simulink model "Discrete_Bicycle_Simulink_Model"  (R2024a)
settings: Solver=ode4  StartTime=0.0  StopTime=100  FixedStep=0.01  RelTol=1e-3
undefined symbols (not defined in the file): Ad, Aobs, Bd, Bobs, c, Cd, Cobs, Dd, Dobs, Kd, lambda, Ts, v, w, x0, xhat0
settings Model: Creator=Vipuls  LastModifiedBy=Vipuls

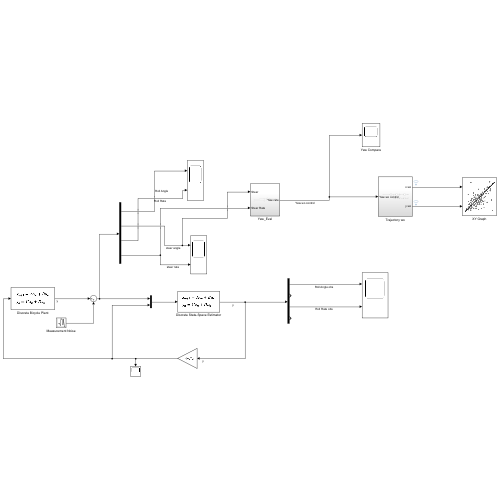
[thumbnail: Simulink's stored preview of the top-level diagram]
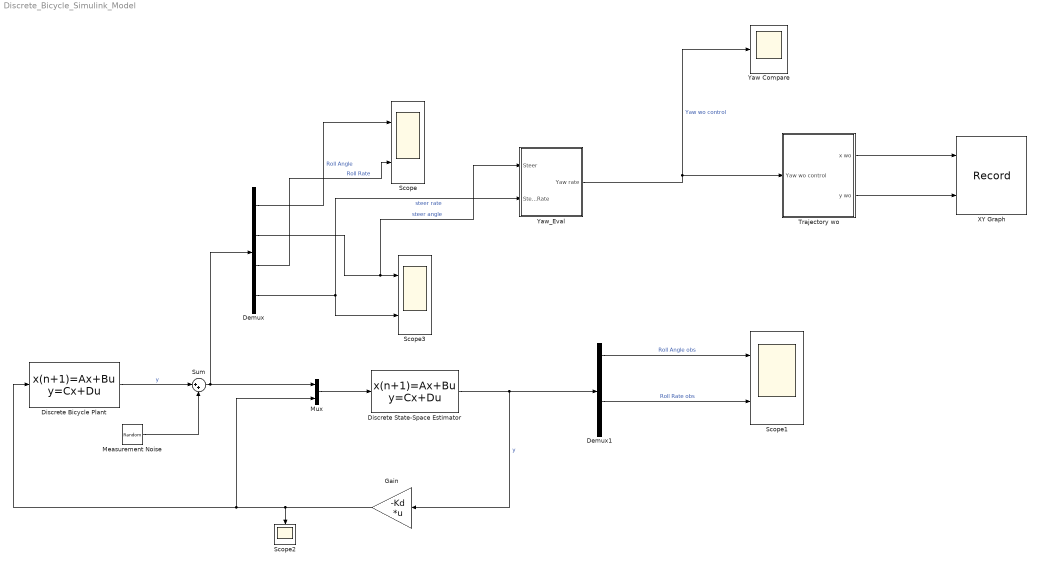
== system Discrete_Bicycle_Simulink_Model ==
  Demux : Demux
  Demux1 : Demux
  Discrete Bicycle Plant : DiscreteStateSpace  A=Ad  B=Bd  C=Cd  D=Dd  InitialCondition=x0  SampleTime=Ts
  Discrete State-Space Estimator : DiscreteStateSpace  A=Aobs  B=Bobs  C=Cobs  D=Dobs  InitialCondition=xhat0  SampleTime=-1
  Gain : Gain  Gain=-Kd  Multiplication=Matrix(K*u)
  Measurement Noise : RandomNumber  Variance=[0.0001, 0.0001, 0.0001, 0.0001]  SampleTime=Ts
  Mux : Mux  Inputs=2
  Scope : Scope  NumInputPorts=2
  Scope1 : Scope  NumInputPorts=2
  Scope2 : Scope
  Scope3 : Scope  NumInputPorts=2
  Sum : Sum  Inputs=|++
  Trajectory wo : Subsystem
  XY Graph : Record  FileSettingsInternal="{\"entries\":[{\"content\":{\"excelSettings\":{\"content\":{},\"type\":\"Streamout.ExcelSettings\"}},\"type\":\"Streamout.FileSettingStorage\",\"uuid\":\"\"}],\"packageUris\":[\"http:\\/\\/schema.mathworks.com\\/mf0\\/streamout_blocks\\/R2020a\"],\"version\":\"1.0\"}"  Layout=[1 1]  SignalsInternal="{\"entries\":[{\"content\":{\"signals\":[{\"content\":{\"blockPath\":[],\"dimensions\":[1],\"domain\":\"\",\"lineColor\":\"#0072bd\",\"lineWidth\":2,\"plots\":[ 1 ],\"port\":1,\"sid\":[\"\"],\"signalID\":1,\"signalName\":\"Trajectory wo:1\"},\"type\":\"RecordBlkView.Signal\",\"uuid\":\"\"},{\"content\":{\"blockPath\":[],\"dimensions\":[1],\"domain\":\"\",\"lineColor\":\"#d95319\",\"lineWidth\":2,\"plots\":[ 1 ],\"port\":2,\"sid\":[\"\"],\"signalID\":2,\"signalName\":\"Trajectory wo:2\"},\"type\":\"RecordBlkView.Signal\",\"uuid\":\"\"}]},\"type\":\"RecordBlkView.InputSignals\",\"uuid\":\"\"}],\"packageUris\":[\"http:\\/\\/schema.mathworks.com\\/mf0\\/streamout_blocks\\/R2020a\"],\"version\":\"1.0\"}"  VisualizationBindings="{\"xyplotplugin\":{\"info\":[{\"series\":[{\"bindingParametersList\":[{\"parameter\":\"X-Axis\",\"signalID\":1,\"signalName\":\"Trajectory wo:1\"},{\"parameter\":\"Y-Axis\",\"signalID\":2,\"signalName\":\"Trajectory wo:2\"}],\"seriesID\":0}],\"subplotID\":1}]}}"  CompatibilityTag=XY
  Yaw Compare : Scope
  Yaw_Eval : Subsystem
  wires:
  Measurement Noise/1 -> Sum/2
  Sum/1 -> Mux/1, Demux/1
  Mux/1 -> Discrete State-Space Estimator/1
  Gain/1 -> Discrete Bicycle Plant/1, Mux/2, Scope2/1
  Demux/1 -> Scope/1  "Roll Angle"
  Demux/3 -> Scope/2  "Roll Rate"
  Discrete State-Space Estimator/1 -> Gain/1, Demux1/1  "y"
  Demux1/3 -> Scope1/2  "Roll Rate obs"
  Demux1/1 -> Scope1/1  "Roll Angle obs"
  Discrete Bicycle Plant/1 -> Sum/1  "y"
  Demux/2 -> Yaw_Eval/1(Steer), Scope3/1  "steer angle"
  Demux/4 -> Scope3/2, Yaw_Eval/2(Steer Rate)  "steer rate"
  Yaw_Eval/1(Yaw rate) -> Trajectory wo/1(Yaw wo control), Yaw Compare/1  "Yaw wo control"
  Trajectory wo/2(y wo) -> XY Graph/2
  Trajectory wo/1(x wo) -> XY Graph/1

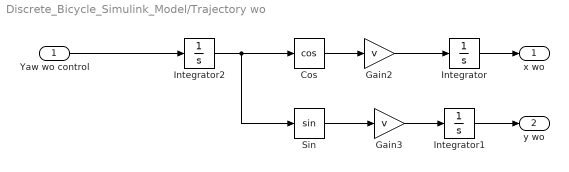
== system Discrete_Bicycle_Simulink_Model/Trajectory wo ==
  Yaw wo control : Inport
  Cos : Trigonometry  Operator=cos
  Gain2 : Gain  Gain=v
  Gain3 : Gain  Gain=v
  Integrator : Integrator
  Integrator1 : Integrator
  Integrator2 : Integrator
  Sin : Trigonometry
  x wo : Outport
  y wo : Outport  Port=2
  wires:
  Sin/1 -> Gain3/1
  Cos/1 -> Gain2/1
  Gain3/1 -> Integrator1/1
  Gain2/1 -> Integrator/1
  Integrator/1 -> x wo/1
  Integrator1/1 -> y wo/1
  Yaw wo control/1 -> Integrator2/1
  Integrator2/1 -> Sin/1, Cos/1

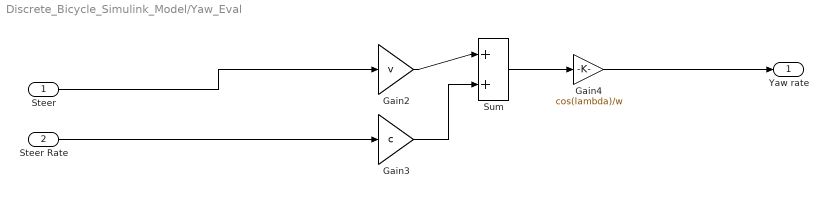
== system Discrete_Bicycle_Simulink_Model/Yaw_Eval ==
  Steer : Inport
  Steer Rate : Inport  Port=2
  Gain2 : Gain  Gain=v
  Gain3 : Gain  Gain=c
  Gain4 : Gain  Gain=cos(lambda)/w
  Sum : Sum  Inputs=|++
  Yaw rate : Outport
  wires:
  Sum/1 -> Gain4/1
  Gain4/1 -> Yaw rate/1
  Gain3/1 -> Sum/2
  Steer Rate/1 -> Gain3/1
  Gain2/1 -> Sum/1
  Steer/1 -> Gain2/1
